simulink model "LAB2D"  (R2020a)
settings: Solver=ode45  StartTime=0.0  StopTime=1  RelTol=1e-3  EnableMultiTasking=on
values from neighbouring files (symbols this model uses):
  D = 0.002    [LAB2.m]
  J = 0.05    [LAB2.m]
  La = 0.03    [LAB2.m]
  psim = 1.1    [LAB2.m]
  Ra = 3    [LAB2.m]
  Ts = 0.0002    [LAB2.m]
  U = 100    [LAB2.m]
  Udc = 600    [LAB2.m]
settings Model: Creator=ielolof  LastModifiedBy=98all
settings DataIOCC: SaveFormat=Array  SignalLoggingSaveFormat=ModelDataLogs  ReturnWorkspaceOutputs=off  TimeSaveName=tpwm
settings OptimizationCC: ExpressionDepthLimit=2147483647  InitFltsAndDblsToZero=on  LifeSpan=inf
settings DebuggingCC: UnderspecifiedInitializationDetection=Classic  MergeDetectMultiDrivingBlocksExec=none  SolverPrmCheckMsg=warning  FcnCallInpInsideContextMsg=warning  StateNameClashWarn=warning  SFUnexpectedBacktrackingDiag=warning  SFNoUnconditionalDefaultTransitionDiag=warning  SFExecutionAtInitializationDiag=none  ArithmeticOperatorsInVariantConditions=warning
settings HardwareCC: ProdBitPerPointer=32  ProdBitPerSizeT=32  ProdBitPerPtrDiffT=32  ProdLargestAtomicFloat=None  ProdIntDivRoundTo=Undefined  ProdEndianess=Unspecified  ProdWordSize=32  ProdHWDeviceType=32-bit Generic
settings ModelReferenceCC: PropagateSignalLabelsOutOfModel=off
settings SFSimCC: SimUseLocalCustomCode=off  CustomCodeUndefinedFunction=UseInterfaceOnly
settings RTWCC: RTWUseLocalCustomCode=off
settings CodeAppCC: StateflowObjectComments=on
settings GRTTargetCC: TargetLangStandard=C89/C90 (ANSI)  CombineOutputUpdateFcns=off  GRTInterface=on
settings ConfigComp: CovMetricSettings=dw  CovHtmlReporting=on  CovSaveCumulativeToWorkspaceVar=on  CovSaveSingleToWorkspaceVar=on  CovExternalEMLEnable=off

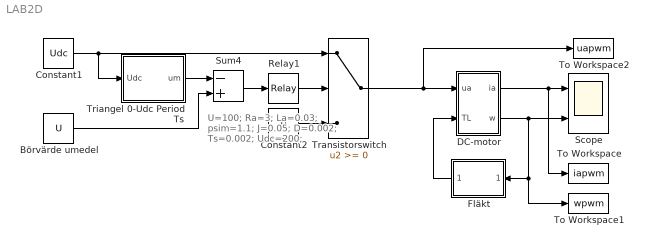
== system LAB2D ==
  note: U=100;
      | Ra=3;
      | La=0.03;
      | psim=1.1;
      | J=0.05;
      | D=0.002;
      |
      | Ts=0.002;
      | Udc=200;
  Börvärde umedel : Constant  Value=U
  Constant1 : Constant  Value=Udc
  Constant2 : Constant  Value=0
  DC-motor : Subsystem
  Fläkt : Subsystem
  Relay1 : Relay  OffOutputValue=-1
  Scope : Scope  NumInputPorts=2
  Sum4 : Sum  Inputs=-+  InputSameDT=on  SaturateOnIntegerOverflow=on  OutDataTypeStr=Inherit: Same as first input
  To Workspace : ToWorkspace  VariableName=iapwm  SampleTime=-1
  To Workspace1 : ToWorkspace  VariableName=wpwm  SampleTime=-1
  To Workspace2 : ToWorkspace  VariableName=uapwm  SampleTime=-1
  Transistorswitch : Switch  SaturateOnIntegerOverflow=on  InputSameDT=on
  Triangel 0-Udc Period Ts : Subsystem
  wires:
  Constant1/1 -> Transistorswitch/1, Triangel 0-Udc Period Ts/1(Udc)
  Constant2/1 -> Transistorswitch/3
  Börvärde umedel/1 -> Sum4/2
  Sum4/1 -> Relay1/1
  Relay1/1 -> Transistorswitch/2
  Triangel 0-Udc Period Ts/1(um) -> Sum4/1
  DC-motor/1(ia) -> Scope/1, To Workspace/1
  DC-motor/2(w) -> Scope/2, Fläkt/1(wfan), To Workspace1/1
  Fläkt/1(Tfan) -> DC-motor/2(TL)
  Transistorswitch/1 -> DC-motor/1(ua), To Workspace2/1

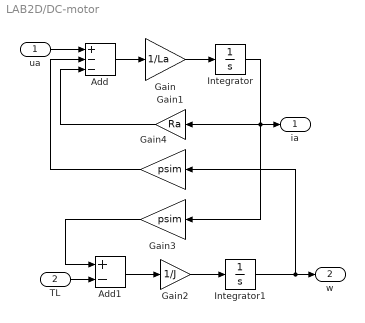
== system LAB2D/DC-motor ==
  ua : Inport
  TL : Inport  Port=2
  Add : Sum  Inputs=+--
  Add1 : Sum  Inputs=+-
  Gain : Gain  Gain=1/La
  Gain1 : Gain  Gain=Ra
  Gain2 : Gain  Gain=1/J
  Gain3 : Gain  Gain=psim
  Gain4 : Gain  Gain=psim
  Integrator : Integrator
  Integrator1 : Integrator
  ia : Outport  VectorParamsAs1DForOutWhenUnconnected=off
  w : Outport  Port=2  VectorParamsAs1DForOutWhenUnconnected=off
  wires:
  Add/1 -> Gain/1
  Gain/1 -> Integrator/1
  Integrator/1 -> Gain1/1, Gain3/1, ia/1
  Add1/1 -> Gain2/1
  Gain2/1 -> Integrator1/1
  Gain3/1 -> Add1/1
  Integrator1/1 -> w/1, Gain4/1
  Gain1/1 -> Add/3
  Gain4/1 -> Add/2
  ua/1 -> Add/1
  TL/1 -> Add1/2

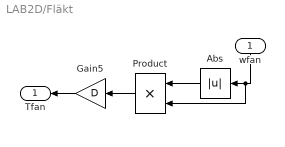
== system LAB2D/Fläkt ==
  wfan : Inport
  Abs : Abs
  Gain5 : Gain  Gain=D
  Product : Product  RndMeth=Zero
  Tfan : Outport  VectorParamsAs1DForOutWhenUnconnected=off
  wires:
  Product/1 -> Gain5/1
  Abs/1 -> Product/1
  wfan/1 -> Abs/1, Product/2
  Gain5/1 -> Tfan/1

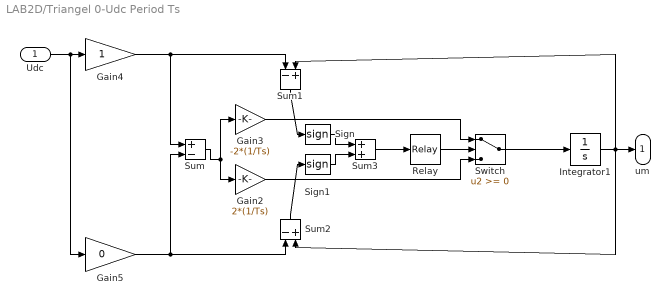
== system LAB2D/Triangel 0-Udc Period Ts ==
  Udc : Inport
  Gain2 : Gain  Gain=2*(1/Ts)  SaturateOnIntegerOverflow=on  OutDataTypeStr=Inherit: Same as input  ParamDataTypeStr=Inherit: Same as input
  Gain3 : Gain  Gain=-2*(1/Ts)  SaturateOnIntegerOverflow=on  OutDataTypeStr=Inherit: Same as input  ParamDataTypeStr=Inherit: Same as input
  Gain4 : Gain  SaturateOnIntegerOverflow=on  OutDataTypeStr=Inherit: Same as input  ParamDataTypeStr=Inherit: Same as input
  Gain5 : Gain  Gain=0  SaturateOnIntegerOverflow=on  OutDataTypeStr=Inherit: Same as input  ParamDataTypeStr=Inherit: Same as input
  Integrator1 : Integrator
  Relay : Relay  OnSwitchValue=1  OffSwitchValue=-1  OffOutputValue=-1
  Sign : Signum
  Sign1 : Signum
  Sum : Sum  Inputs=+-  InputSameDT=on  SaturateOnIntegerOverflow=on  OutDataTypeStr=Inherit: Same as first input
  Sum1 : Sum  Inputs=-+  InputSameDT=on  SaturateOnIntegerOverflow=on  OutDataTypeStr=Inherit: Same as first input
  Sum2 : Sum  Inputs=-+  InputSameDT=on  SaturateOnIntegerOverflow=on  OutDataTypeStr=Inherit: Same as first input
  Sum3 : Sum  InputSameDT=on  SaturateOnIntegerOverflow=on  OutDataTypeStr=Inherit: Same as first input
  Switch : Switch  SaturateOnIntegerOverflow=on  InputSameDT=on
  um : Outport  VectorParamsAs1DForOutWhenUnconnected=off
  wires:
  Switch/1 -> Integrator1/1
  Gain3/1 -> Switch/1
  Gain2/1 -> Switch/3
  Integrator1/1 -> Sum1/2, Sum2/2, um/1
  Sum1/1 -> Sign/1
  Sum2/1 -> Sign1/1
  Sign/1 -> Sum3/1
  Sign1/1 -> Sum3/2
  Sum3/1 -> Relay/1
  Relay/1 -> Switch/2
  Sum/1 -> Gain3/1, Gain2/1
  Udc/1 -> Gain5/1, Gain4/1
  Gain5/1 -> Sum/2, Sum2/1
  Gain4/1 -> Sum/1, Sum1/1
